simulink model "inverse_model"  (R2019a)
settings: Solver=VariableStepAuto  StartTime=0.0  StopTime=10.0  RelTol=1e-3

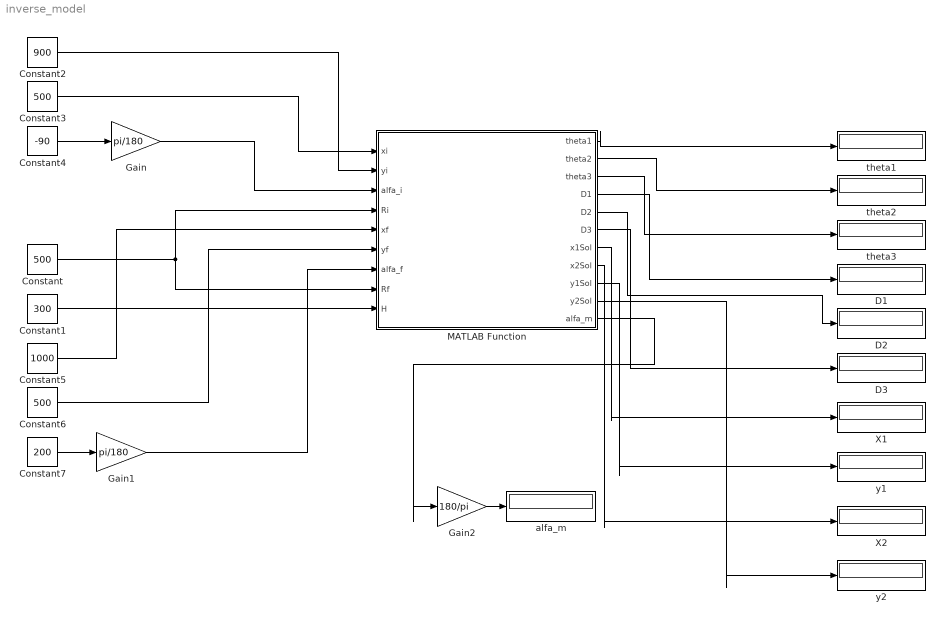
== system inverse_model ==
  Constant : Constant  Value=500
  Constant1 : Constant  Value=300
  Constant2 : Constant  Value=900
  Constant3 : Constant  Value=500
  Constant4 : Constant  Value=-90
  Constant5 : Constant  Value=1000
  Constant6 : Constant  Value=500
  Constant7 : Constant  Value=200
  D1 : Display
  D2 : Display
  D3 : Display
  Gain : Gain  Gain=pi/180
  Gain1 : Gain  Gain=pi/180
  Gain2 : Gain  Gain=180/pi
  MATLAB Function : MATLAB Function  TreatAsAtomicUnit=on
  X1 : Display
  X2 : Display
  alfa_m : Display
  theta1 : Display
  theta2 : Display
  theta3 : Display
  y1 : Display
  y2 : Display
  wires:
  Constant/1 -> MATLAB Function/4(Ri), MATLAB Function/8(Rf)
  Constant1/1 -> MATLAB Function/9(H)
  Constant2/1 -> MATLAB Function/2(yi)
  Constant3/1 -> MATLAB Function/1(xi)
  Constant4/1 -> Gain/1
  Gain/1 -> MATLAB Function/3(alfa_i)
  Constant5/1 -> MATLAB Function/5(xf)
  Constant6/1 -> MATLAB Function/6(yf)
  Constant7/1 -> Gain1/1
  Gain1/1 -> MATLAB Function/7(alfa_f)
  MATLAB Function/1(theta1) -> theta1/1
  MATLAB Function/2(theta2) -> theta2/1
  MATLAB Function/3(theta3) -> theta3/1
  MATLAB Function/4(D1) -> D1/1
  MATLAB Function/5(D2) -> D2/1
  MATLAB Function/6(D3) -> D3/1
  MATLAB Function/7(x1Sol) -> X1/1
  MATLAB Function/8(x2Sol) -> X2/1
  MATLAB Function/9(y1Sol) -> y1/1
  MATLAB Function/10(y2Sol) -> y2/1
  MATLAB Function/11(alfa_m) -> Gain2/1
  Gain2/1 -> alfa_m/1

== matlab function inverse_model/MATLAB Function ==
function [theta1,theta2,theta3,D1,D2,D3,x1Sol,x2Sol,y1Sol,y2Sol,alfa_m] = fcn(xi,yi,alfa_i,Ri,xf,yf,alfa_f,Rf,H)


%H=200;
%Ri=500;Rf=500;
%xi=5000; yi=5000; alfa_i=90*pi/180;
%xf=0; yf=0; alfa_f=0*pi/180;


xc1=xf+Rf*sin(alfa_f);
yc1=yf-Rf*cos(alfa_f);
xc2=xi+Ri*sin(alfa_i);
yc2=yi-Ri*cos(alfa_i);

%v1=[(x1-xc1),(y1-yc1),0];
%v2=[(x1-x2),(y1-y2)],0;
%v3=[(x2-xc2),(y2-yc2),0];

%syms x1 y1 x2 y2 xc1 xc2 yc1 yc2 Rf Ri
%eqn1 = ((x1-xc1)*(x1-x2)+(y1-yc1)*(y1-y2)) == 0;
%eqn2 = ((x1 - xc1)*(y2 - yc2) - (x2 - xc2)*(y1 - yc1)) == 0;
%eqn3 = (x1-xc1)^2 + (y1-yc1)^2 == (Rf)^2;
%eqn4 = (x2-xc2)^2 + (y2-yc2)^2 == (Ri)^2;

%sol = solve([eqn1, eqn2, eqn3, eqn4], [x1, y1, x2, y2]);
%x1Sol = sol.x1
%y1Sol = sol.y1
%x2Sol = sol.x2
%y2Sol = sol.y2


x1Sol =(- Rf^2*Ri + Rf*Ri^2 - Rf*yc2^2 + yc1*Rf*yc2 + Ri*xc1^2 -xc2*Ri*xc1)/(Ri*(xc1 - xc2)) - ((Rf*yc1 - Rf*yc2)*(Ri^2*yc1 - Ri^2*yc2 + xc1^2*yc2 + xc2^2*yc2 - 2*yc1*yc2^2 + yc1^2*yc2 + yc2^3 + Ri*xc1*(- Rf^2 + 2*Rf*Ri - Ri^2 + xc1^2 - 2*xc1*xc2 + xc2^2 + yc1^2 - 2*yc1*yc2 + yc2^2)^(1/2) - Ri*xc2*(- Rf^2 + 2*Rf*Ri - Ri^2 + xc1^2 - 2*xc1*xc2 + xc2^2 + yc1^2 - 2*yc1*yc2 + yc2^2)^(1/2) - Rf*Ri*yc1 + Rf*Ri*yc2 - 2*xc1*xc2*yc2))/(Ri*(xc1 - xc2)*(xc1^2 - 2*xc1*xc2 + xc2^2 + yc1^2 - 2*yc1*yc2 + yc2^2));
 
%((Rf*yc1 - Rf*yc2)*(Ri^2*yc1 - Ri^2*yc2 + xc1^2*yc2 + xc2^2*yc2 - 2*yc1*yc2^2 + yc1^2*yc2 + yc2^3 + Ri*xc1*(- Rf^2 - 2*Rf*Ri - Ri^2 + xc1^2 - 2*xc1*xc2 + xc2^2 + yc1^2 - 2*yc1*yc2 + yc2^2)^(1/2) - Ri*xc2*(- Rf^2 - 2*Rf*Ri - Ri^2 + xc1^2 - 2*xc1*xc2 + xc2^2 + yc1^2 - 2*yc1*yc2 + yc2^2)^(1/2) + Rf*Ri*yc1 - Rf*Ri*yc2 - 2*xc1*xc2*yc2))/(Ri*(xc1 - xc2)*(xc1^2 - 2*xc1*xc2 + xc2^2 + yc1^2 - 2*yc1*yc2 + yc2^2)) - (Rf^2*Ri + Rf*Ri^2 - Rf*yc2^2 + yc1*Rf*yc2 - Ri*xc1^2 + xc2*Ri*xc1)/(Ri*(xc1 - xc2));
  
% ((Rf*yc1 - Rf*yc2)*(Ri^2*yc1 - Ri^2*yc2 + xc1^2*yc2 + xc2^2*yc2 - 2*yc1*yc2^2 + yc1^2*yc2 + yc2^3 - Ri*xc1*(- Rf^2 - 2*Rf*Ri - Ri^2 + xc1^2 - 2*xc1*xc2 + xc2^2 + yc1^2 - 2*yc1*yc2 + yc2^2)^(1/2) + Ri*xc2*(- Rf^2 - 2*Rf*Ri - Ri^2 + xc1^2 - 2*xc1*xc2 + xc2^2 + yc1^2 - 2*yc1*yc2 + yc2^2)^(1/2) + Rf*Ri*yc1 - Rf*Ri*yc2 - 2*xc1*xc2*yc2))/(Ri*(xc1 - xc2)*(xc1^2 - 2*xc1*xc2 + xc2^2 + yc1^2 - 2*yc1*yc2 + yc2^2)) - (Rf^2*Ri + Rf*Ri^2 - Rf*yc2^2 + yc1*Rf*yc2 - Ri*xc1^2 + xc2*Ri*xc1)/(Ri*(xc1 - xc2));
 
%(- Rf^2*Ri + Rf*Ri^2 - Rf*yc2^2 + yc1*Rf*yc2 + Ri*xc1^2 -xc2*Ri*xc1)/(Ri*(xc1 - xc2)) - ((Rf*yc1 - Rf*yc2)*(Ri^2*yc1 - Ri^2*yc2 + xc1^2*yc2 + xc2^2*yc2 - 2*yc1*yc2^2 + yc1^2*yc2 + yc2^3 + Ri*xc1*(- Rf^2 + 2*Rf*Ri - Ri^2 + xc1^2 - 2*xc1*xc2 + xc2^2 + yc1^2 - 2*yc1*yc2 + yc2^2)^(1/2) - Ri*xc2*(- Rf^2 + 2*Rf*Ri - Ri^2 + xc1^2 - 2*xc1*xc2 + xc2^2 + yc1^2 - 2*yc1*yc2 + yc2^2)^(1/2) - Rf*Ri*yc1 + Rf*Ri*yc2 - 2*xc1*xc2*yc2))/(Ri*(xc1 - xc2)*(xc1^2 - 2*xc1*xc2 + xc2^2 + yc1^2 - 2*yc1*yc2 + yc2^2));
 
%(- Rf^2*Ri + Rf*Ri^2 - Rf*yc2^2 + yc1*Rf*yc2 + Ri*xc1^2 -xc2*Ri*xc1)/(Ri*(xc1 - xc2)) - ((Rf*yc1 - Rf*yc2)*(Ri^2*yc1 - Ri^2*yc2 + xc1^2*yc2 + xc2^2*yc2 - 2*yc1*yc2^2 + yc1^2*yc2 + yc2^3 - Ri*xc1*(- Rf^2 + 2*Rf*Ri - Ri^2 + xc1^2 - 2*xc1*xc2 + xc2^2 + yc1^2 - 2*yc1*yc2 + yc2^2)^(1/2) + Ri*xc2*(- Rf^2 + 2*Rf*Ri - Ri^2 + xc1^2 - 2*xc1*xc2 + xc2^2 + yc1^2 - 2*yc1*yc2 + yc2^2)^(1/2) - Rf*Ri*yc1 + Rf*Ri*yc2 - 2*xc1*xc2*yc2))/(Ri*(xc1 - xc2)*(xc1^2 - 2*xc1*xc2 + xc2^2 + yc1^2 - 2*yc1*yc2 + yc2^2));
 
 
y1Sol =(Ri*yc1 - Rf*yc2 + (Rf*(Ri^2*yc1 - Ri^2*yc2 + xc1^2*yc2 + xc2^2*yc2 -2*yc1*yc2^2 + yc1^2*yc2 + yc2^3 + Ri*xc1*(- Rf^2 + 2*Rf*Ri - Ri^2 + xc1^2 - 2*xc1*xc2 + xc2^2 + yc1^2 - 2*yc1*yc2 + yc2^2)^(1/2) - Ri*xc2*(- Rf^2 + 2*Rf*Ri - Ri^2 + xc1^2 - 2*xc1*xc2 + xc2^2 + yc1^2 - 2*yc1*yc2 + yc2^2)^(1/2) - Rf*Ri*yc1 + Rf*Ri*yc2 - 2*xc1*xc2*yc2))/(xc1^2 - 2*xc1*xc2 + xc2^2 + yc1^2 - 2*yc1*yc2 + yc2^2))/Ri;


%(Rf*yc2 + Ri*yc1 - (Rf*(Ri^2*yc1 - Ri^2*yc2 + xc1^2*yc2 + xc2^2*yc2 - 2*yc1*yc2^2 + yc1^2*yc2 + yc2^3 + Ri*xc1*(- Rf^2 - 2*Rf*Ri - Ri^2 + xc1^2 - 2*xc1*xc2 + xc2^2 + yc1^2 - 2*yc1*yc2 + yc2^2)^(1/2) - Ri*xc2*(- Rf^2 - 2*Rf*Ri - Ri^2 + xc1^2 - 2*xc1*xc2 + xc2^2 + yc1^2 - 2*yc1*yc2 + yc2^2)^(1/2) + Rf*Ri*yc1 - Rf*Ri*yc2 - 2*xc1*xc2*yc2))/(xc1^2 - 2*xc1*xc2 + xc2^2 + yc1^2 - 2*yc1*yc2 + yc2^2))/Ri;

%(Rf*yc2 + Ri*yc1 - (Rf*(Ri^2*yc1 - Ri^2*yc2 + xc1^2*yc2 + xc2^2*yc2 -2*yc1*yc2^2 + yc1^2*yc2 + yc2^3 - Ri*xc1*(- Rf^2 - 2*Rf*Ri - Ri^2 + xc1^2 - 2*xc1*xc2 + xc2^2 + yc1^2 - 2*yc1*yc2 + yc2^2)^(1/2) + Ri*xc2*(- Rf^2 - 2*Rf*Ri - Ri^2 + xc1^2 - 2*xc1*xc2 + xc2^2 + yc1^2 - 2*yc1*yc2 + yc2^2)^(1/2) + Rf*Ri*yc1 - Rf*Ri*yc2 - 2*xc1*xc2*yc2))/(xc1^2 - 2*xc1*xc2 + xc2^2 + yc1^2 - 2*yc1*yc2 + yc2^2))/Ri;

%(Ri*yc1 - Rf*yc2 + (Rf*(Ri^2*yc1 - Ri^2*yc2 + xc1^2*yc2 + xc2^2*yc2 -2*yc1*yc2^2 + yc1^2*yc2 + yc2^3 + Ri*xc1*(- Rf^2 + 2*Rf*Ri - Ri^2 + xc1^2 - 2*xc1*xc2 + xc2^2 + yc1^2 - 2*yc1*yc2 + yc2^2)^(1/2) - Ri*xc2*(- Rf^2 + 2*Rf*Ri - Ri^2 + xc1^2 - 2*xc1*xc2 + xc2^2 + yc1^2 - 2*yc1*yc2 + yc2^2)^(1/2) - Rf*Ri*yc1 + Rf*Ri*yc2 - 2*xc1*xc2*yc2))/(xc1^2 - 2*xc1*xc2 + xc2^2 + yc1^2 - 2*yc1*yc2 + yc2^2))/Ri;
 
%(Ri*yc1 - Rf*yc2 + (Rf*(Ri^2*yc1 - Ri^2*yc2 + xc1^2*yc2 + xc2^2*yc2 -2*yc1*yc2^2 + yc1^2*yc2 + yc2^3 - Ri*xc1*(- Rf^2 + 2*Rf*Ri - Ri^2 + xc1^2 - 2*xc1*xc2 + xc2^2 + yc1^2 - 2*yc1*yc2 + yc2^2)^(1/2) + Ri*xc2*(- Rf^2 + 2*Rf*Ri - Ri^2 + xc1^2 - 2*xc1*xc2 + xc2^2 + yc1^2 - 2*yc1*yc2 + yc2^2)^(1/2) - Rf*Ri*yc1 + Rf*Ri*yc2 - 2*xc1*xc2*yc2))/(xc1^2 - 2*xc1*xc2 + xc2^2 + yc1^2 - 2*yc1*yc2 + yc2^2))/Ri;
 
 
x2Sol = - (- Ri^2 + Rf*Ri + xc2^2 - xc1*xc2 + yc2^2 - yc1*yc2)/(xc1 - xc2) - ((yc1 - yc2)*(Ri^2*yc1 - Ri^2*yc2 + xc1^2*yc2 + xc2^2*yc2 - 2*yc1*yc2^2 + yc1^2*yc2 + yc2^3 + Ri*xc1*(- Rf^2 + 2*Rf*Ri - Ri^2 + xc1^2 - 2*xc1*xc2 + xc2^2 + yc1^2 - 2*yc1*yc2 + yc2^2)^(1/2) - Ri*xc2*(- Rf^2 + 2*Rf*Ri - Ri^2 + xc1^2 - 2*xc1*xc2 + xc2^2 + yc1^2 - 2*yc1*yc2 + yc2^2)^(1/2) - Rf*Ri*yc1 + Rf*Ri*yc2 - 2*xc1*xc2*yc2))/((xc1 - xc2)*(xc1^2 - 2*xc1*xc2 + xc2^2 + yc1^2 - 2*yc1*yc2 + yc2^2));

% (Ri^2 + Rf*Ri - xc2^2 + xc1*xc2 - yc2^2 + yc1*yc2)/(xc1 - xc2) - ((yc1 - yc2)*(Ri^2*yc1 - Ri^2*yc2 + xc1^2*yc2 + xc2^2*yc2 - 2*yc1*yc2^2 + yc1^2*yc2 + yc2^3 + Ri*xc1*(- Rf^2 - 2*Rf*Ri - Ri^2 + xc1^2 - 2*xc1*xc2 + xc2^2 + yc1^2 - 2*yc1*yc2 + yc2^2)^(1/2) - Ri*xc2*(- Rf^2 - 2*Rf*Ri - Ri^2 + xc1^2 - 2*xc1*xc2 + xc2^2 + yc1^2 - 2*yc1*yc2 + yc2^2)^(1/2) + Rf*Ri*yc1 - Rf*Ri*yc2 - 2*xc1*xc2*yc2))/((xc1 - xc2)*(xc1^2 - 2*xc1*xc2 + xc2^2 + yc1^2 - 2*yc1*yc2 + yc2^2));
  
% (Ri^2 + Rf*Ri - xc2^2 + xc1*xc2 - yc2^2 + yc1*yc2)/(xc1 - xc2) - ((yc1 - yc2)*(Ri^2*yc1 - Ri^2*yc2 + xc1^2*yc2 + xc2^2*yc2 - 2*yc1*yc2^2 + yc1^2*yc2 + yc2^3 - Ri*xc1*(- Rf^2 - 2*Rf*Ri - Ri^2 + xc1^2 - 2*xc1*xc2 + xc2^2 + yc1^2 - 2*yc1*yc2 + yc2^2)^(1/2) + Ri*xc2*(- Rf^2 - 2*Rf*Ri - Ri^2 + xc1^2 - 2*xc1*xc2 + xc2^2 + yc1^2 - 2*yc1*yc2 + yc2^2)^(1/2) + Rf*Ri*yc1 - Rf*Ri*yc2 - 2*xc1*xc2*yc2))/((xc1 - xc2)*(xc1^2 - 2*xc1*xc2 + xc2^2 + yc1^2 - 2*yc1*yc2 + yc2^2));

% - (- Ri^2 + Rf*Ri + xc2^2 - xc1*xc2 + yc2^2 - yc1*yc2)/(xc1 - xc2) - ((yc1 - yc2)*(Ri^2*yc1 - Ri^2*yc2 + xc1^2*yc2 + xc2^2*yc2 - 2*yc1*yc2^2 + yc1^2*yc2 + yc2^3 + Ri*xc1*(- Rf^2 + 2*Rf*Ri - Ri^2 + xc1^2 - 2*xc1*xc2 + xc2^2 + yc1^2 - 2*yc1*yc2 + yc2^2)^(1/2) - Ri*xc2*(- Rf^2 + 2*Rf*Ri - Ri^2 + xc1^2 - 2*xc1*xc2 + xc2^2 + yc1^2 - 2*yc1*yc2 + yc2^2)^(1/2) - Rf*Ri*yc1 + Rf*Ri*yc2 - 2*xc1*xc2*yc2))/((xc1 - xc2)*(xc1^2 - 2*xc1*xc2 + xc2^2 + yc1^2 - 2*yc1*yc2 + yc2^2));

% - (- Ri^2 + Rf*Ri + xc2^2 - xc1*xc2 + yc2^2 - yc1*yc2)/(xc1 - xc2) - ((yc1 - yc2)*(Ri^2*yc1 - Ri^2*yc2 + xc1^2*yc2 + xc2^2*yc2 - 2*yc1*yc2^2 + yc1^2*yc2 + yc2^3 - Ri*xc1*(- Rf^2 + 2*Rf*Ri - Ri^2 + xc1^2 - 2*xc1*xc2 + xc2^2 + yc1^2 - 2*yc1*yc2 + yc2^2)^(1/2) + Ri*xc2*(- Rf^2 + 2*Rf*Ri - Ri^2 + xc1^2 - 2*xc1*xc2 + xc2^2 + yc1^2 - 2*yc1*yc2 + yc2^2)^(1/2) - Rf*Ri*yc1 + Rf*Ri*yc2 - 2*xc1*xc2*yc2))/((xc1 - xc2)*(xc1^2 - 2*xc1*xc2 + xc2^2 + yc1^2 - 2*yc1*yc2 + yc2^2));
 
 
y2Sol =(Ri^2*yc1 - Ri^2*yc2 + xc1^2*yc2 + xc2^2*yc2 - 2*yc1*yc2^2 + yc1^2*yc2 + yc2^3 + Ri*xc1*(- Rf^2 + 2*Rf*Ri - Ri^2 + xc1^2 - 2*xc1*xc2 + xc2^2 + yc1^2 - 2*yc1*yc2 + yc2^2)^(1/2) - Ri*xc2*(- Rf^2 + 2*Rf*Ri - Ri^2 + xc1^2 - 2*xc1*xc2 + xc2^2 + yc1^2 - 2*yc1*yc2 + yc2^2)^(1/2) - Rf*Ri*yc1 + Rf*Ri*yc2 - 2*xc1*xc2*yc2)/(xc1^2 - 2*xc1*xc2 + xc2^2 + yc1^2 - 2*yc1*yc2 + yc2^2);
 
%(Ri^2*yc1 - Ri^2*yc2 + xc1^2*yc2 + xc2^2*yc2 - 2*yc1*yc2^2 + yc1^2*yc2 + yc2^3 + Ri*xc1*(- Rf^2 - 2*Rf*Ri - Ri^2 + xc1^2 - 2*xc1*xc2 + xc2^2 + yc1^2 - 2*yc1*yc2 + yc2^2)^(1/2) - Ri*xc2*(- Rf^2 - 2*Rf*Ri - Ri^2 + xc1^2 - 2*xc1*xc2 + xc2^2 + yc1^2 - 2*yc1*yc2 + yc2^2)^(1/2) + Rf*Ri*yc1 - Rf*Ri*yc2 - 2*xc1*xc2*yc2)/(xc1^2 - 2*xc1*xc2 + xc2^2 + yc1^2 - 2*yc1*yc2 + yc2^2);
 
%(Ri^2*yc1 - Ri^2*yc2 + xc1^2*yc2 + xc2^2*yc2 - 2*yc1*yc2^2 + yc1^2*yc2 +yc2^3 - Ri*xc1*(- Rf^2 - 2*Rf*Ri - Ri^2 + xc1^2 - 2*xc1*xc2 + xc2^2 + yc1^2 - 2*yc1*yc2 + yc2^2)^(1/2) + Ri*xc2*(- Rf^2 - 2*Rf*Ri - Ri^2 + xc1^2 - 2*xc1*xc2 + xc2^2 + yc1^2 - 2*yc1*yc2 + yc2^2)^(1/2) + Rf*Ri*yc1 - Rf*Ri*yc2 - 2*xc1*xc2*yc2)/(xc1^2 - 2*xc1*xc2 + xc2^2 + yc1^2 - 2*yc1*yc2 + yc2^2);
 
%(Ri^2*yc1 - Ri^2*yc2 + xc1^2*yc2 + xc2^2*yc2 - 2*yc1*yc2^2 + yc1^2*yc2 + yc2^3 + Ri*xc1*(- Rf^2 + 2*Rf*Ri - Ri^2 + xc1^2 - 2*xc1*xc2 + xc2^2 + yc1^2 - 2*yc1*yc2 + yc2^2)^(1/2) - Ri*xc2*(- Rf^2 + 2*Rf*Ri - Ri^2 + xc1^2 - 2*xc1*xc2 + xc2^2 + yc1^2 - 2*yc1*yc2 + yc2^2)^(1/2) - Rf*Ri*yc1 + Rf*Ri*yc2 - 2*xc1*xc2*yc2)/(xc1^2 - 2*xc1*xc2 + xc2^2 + yc1^2 - 2*yc1*yc2 + yc2^2);
 
%(Ri^2*yc1 - Ri^2*yc2 + xc1^2*yc2 + xc2^2*yc2 - 2*yc1*yc2^2 + yc1^2*yc2 + yc2^3 - Ri*xc1*(- Rf^2 + 2*Rf*Ri - Ri^2 + xc1^2 - 2*xc1*xc2 + xc2^2 + yc1^2 - 2*yc1*yc2 + yc2^2)^(1/2) + Ri*xc2*(- Rf^2 + 2*Rf*Ri - Ri^2 + xc1^2 - 2*xc1*xc2 + xc2^2 + yc1^2 - 2*yc1*yc2 + yc2^2)^(1/2) - Rf*Ri*yc1 + Rf*Ri*yc2 - 2*xc1*xc2*yc2)/(xc1^2 - 2*xc1*xc2 + xc2^2 + yc1^2 - 2*yc1*yc2 + yc2^2);

d2x1=cos(alfa_i);
d2y1=sin(alfa_i);
d2x2=x2Sol-xi;
d2y2=y2Sol-yi;
Cross2=(d2x1*d2y2-d2y1*d2x2);

d1x1=cos(alfa_f);
d1y1=sin(alfa_f);
d1x2=x1Sol-xf;
d1y2=y1Sol-yf;
Cross1=(d1x1*d1y2-d1y1*d1x2);

if (Cross2 > 0)
   sign_1st=-1;
else  
    sign_1st=1;
end 

if (Cross1 > 0)
   sign_2nd=-1;
else  
    sign_2nd=1;
end 

theta1=sign_1st*(90-atand(Ri/H));
theta2=0.000001;
theta3=sign_2nd*(90-atand(Rf/H));

%sign_1st*(90-atand(Ri/H));
%sign_1st*
%sign_2nd*

cosangle1=((y2Sol-yi)*sin(alfa_i)+(x2Sol-xi)*cos(alfa_i));

if (cosangle1 < 0)
   s_1st=-1;
else  
    s_1st=1;
end 

D1=s_1st*Ri*acos((((x2Sol-xc2)*(xi-xc2)+(y2Sol-yc2)*(yi-yc2))/Ri^2)-9e-15);

L=-H/cos((pi/2)-theta1*pi/180);
beta = D1/(L*cos(theta1*pi/180));
alfa_m =  alfa_i + beta;

cosangle2=((y1Sol-y2Sol)*sin(alfa_m)+(x1Sol-x2Sol)*cos(alfa_m));
cosangle3=((yf-y1Sol)*sin(alfa_m)+(xf-x1Sol)*cos(alfa_m));

if (cosangle2 < 0)
   s_2nd=-1;
else  
    s_2nd=1;
end 
if (cosangle3 < 0)
   s_3rd=-1;
else  
    s_3rd=1;
end 



D2=s_2nd*((x1Sol-x2Sol)^2+(y1Sol-y2Sol)^2)^0.5;
D3=s_3rd*Rf*acos((((x1Sol-xc1)*(xf-xc1)+(y1Sol-yc1)*(yf-yc1))/Rf^2)-9e-15);

%s_1st*
%s_1st*s_2nd*
%s_1st*s_2nd*s_3rd*
